simulink model "SCS_check_modified"  (R2022b)
settings: Solver=VariableStepAuto  StartTime=0.0  StopTime=10.0  RelTol=1e-3
libraries: simulink x14
settings Model: Creator=tiszu  LastModifiedBy=tiszu

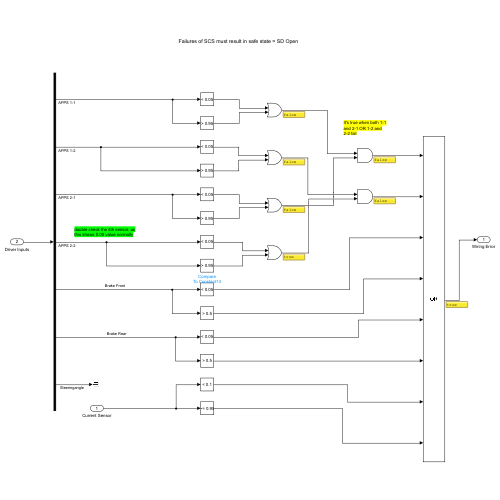
[thumbnail: Simulink's stored preview of the top-level diagram]
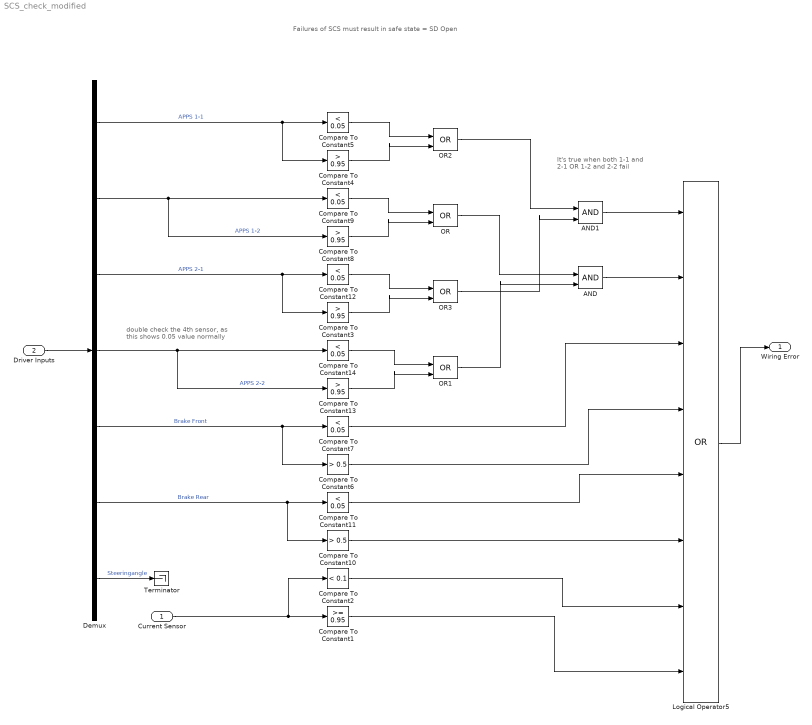
== system SCS_check_modified ==
  note: It's true when both 1-1 and 2-1 OR 1-2 and 2-2 fail
  note: double check the 4th sensor, as this shows 0.05 value normally
  note: Failures of SCS must result in safe state = SD Open
  Current Sensor : Inport
  Driver Inputs : Inport  Port=2
  AND : Logic  IconShape=distinctive  AllPortsSameDT=off  OutDataTypeStr=boolean
  AND1 : Logic  IconShape=distinctive  AllPortsSameDT=off  OutDataTypeStr=boolean
  Compare To Constant1 : simulink/Logic and Bit Operations/Compare To Constant  relop=>=  const=0.95  OutDataTypeStr=boolean
  Compare To Constant10 : simulink/Logic and Bit Operations/Compare To Constant  relop=>  const=0.5  OutDataTypeStr=boolean
  Compare To Constant{5,7,9,11..12,14} (6 alike) : simulink/Logic and Bit Operations/Compare To Constant  relop=<  const=0.05  OutDataTypeStr=boolean
  Compare To Constant{3..4,8,13} (4 alike) : simulink/Logic and Bit Operations/Compare To Constant  relop=>  const=0.95  OutDataTypeStr=boolean
  Compare To Constant2 : simulink/Logic and Bit Operations/Compare To Constant  relop=<  const=0.1  OutDataTypeStr=boolean
  Compare To Constant6 : simulink/Logic and Bit Operations/Compare To Constant  relop=>  const=0.5  OutDataTypeStr=boolean
  Demux : Demux  Outputs=7
  Logical Operator5 : Logic  Operator=OR  Inputs=8  AllPortsSameDT=off  OutDataTypeStr=boolean
  OR{,1..3} (4 alike) : Logic  Operator=OR  IconShape=distinctive  AllPortsSameDT=off  OutDataTypeStr=boolean
  Terminator : Terminator
  Wiring Error : Outport
  wires:
  Demux/1 -> Compare To Constant4/1, Compare To Constant5/1  "APPS 1-1"
  Compare To Constant13/1 -> OR1/2
  Compare To Constant14/1 -> OR1/1
  Compare To Constant9/1 -> OR/1
  Compare To Constant2/1 -> Logical Operator5/7
  Current Sensor/1 -> Compare To Constant2/1, Compare To Constant1/1
  Compare To Constant1/1 -> Logical Operator5/8
  Compare To Constant12/1 -> OR3/1
  Demux/2 -> Compare To Constant8/1, Compare To Constant9/1  "APPS 1-2"
  Demux/5 -> Compare To Constant6/1, Compare To Constant7/1  "Brake Front"
  Demux/4 -> Compare To Constant14/1, Compare To Constant13/1  "APPS 2-2"
  Driver Inputs/1 -> Demux/1
  Compare To Constant8/1 -> OR/2
  Compare To Constant6/1 -> Logical Operator5/4
  Compare To Constant4/1 -> OR2/2
  Compare To Constant10/1 -> Logical Operator5/6
  Compare To Constant7/1 -> Logical Operator5/3
  Logical Operator5/1 -> Wiring Error/1
  Demux/7 -> Terminator/1  "Steeringangle"
  Compare To Constant5/1 -> OR2/1
  Demux/3 -> Compare To Constant3/1, Compare To Constant12/1  "APPS 2-1"
  Demux/6 -> Compare To Constant11/1, Compare To Constant10/1  "Brake Rear"
  Compare To Constant3/1 -> OR3/2
  OR1/1 -> AND/2
  OR/1 -> AND/1
  OR2/1 -> AND1/1
  OR3/1 -> AND1/2
  Compare To Constant11/1 -> Logical Operator5/5
  AND1/1 -> Logical Operator5/1
  AND/1 -> Logical Operator5/2
